simulink model "azmayeshe_AC_source"  (R2015a)
settings: Solver=ode45  StartTime=0.02  StopTime=0.04  RelTol=1e-3
libraries: powerlib x44, simulink x14, powerlib_meascontrol x14
settings Model: Creator=Yahya  LastModifiedBy=Yahya

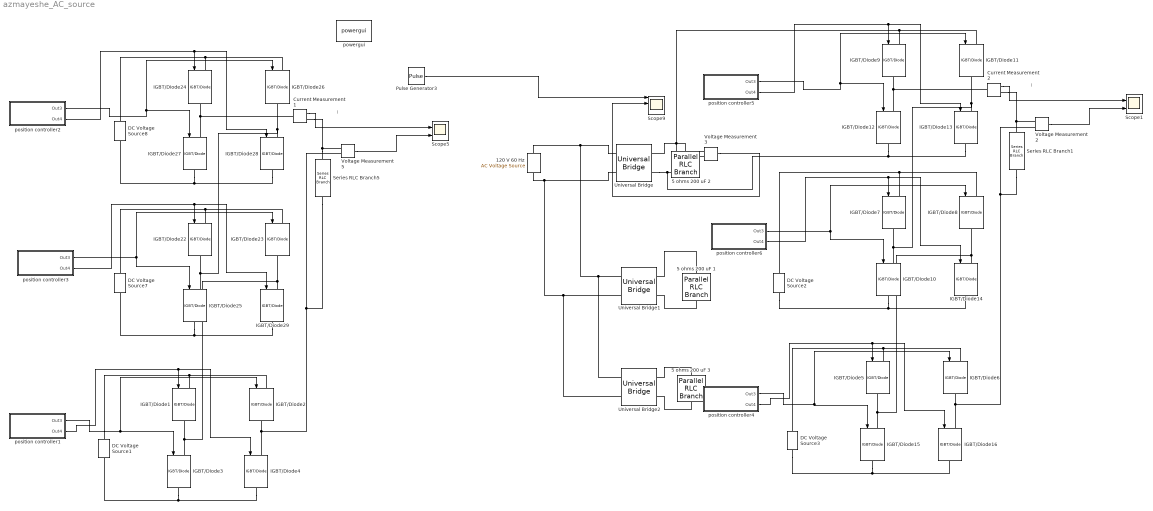
== system azmayeshe_AC_source ==
  note: i
  note: i
  120 V 60 Hz : powerlib/Electrical Sources/AC Voltage Source  Description=source block  Amplitude=100  Phase=0  Frequency=60  SampleTime=0  Measurements=None
      settings: AttributesFormatString=\n
  5 ohms 200 uF 1 : powerlib/Elements/Parallel RLC Branch  LConnTagsString=a  RConnTagsString=__new0  BranchType=C  Resistance=5  Inductance=1.0  SetiL0=off  InitialCurrent=0  Capacitance=470e-06  Setx0=off  InitialVoltage=0  Measurements=None
  5 ohms 200 uF 2 : powerlib/Elements/Parallel RLC Branch  LConnTagsString=a  RConnTagsString=__new0  BranchType=C  Resistance=5  Inductance=1.0  SetiL0=off  InitialCurrent=0  Capacitance=470e-06  Setx0=off  InitialVoltage=0  Measurements=None
  5 ohms 200 uF 3 : powerlib/Elements/Parallel RLC Branch  LConnTagsString=a  RConnTagsString=__new0  BranchType=C  Resistance=5  Inductance=1.0  SetiL0=off  InitialCurrent=0  Capacitance=470e-06  Setx0=off  InitialVoltage=0  Measurements=None
  Current Measurement1 : powerlib/Measurements/Current Measurement  PhasorSimulation=off  OutputType=Complex  PSBequivalent=0
  Current Measurement2 : powerlib/Measurements/Current Measurement  PhasorSimulation=off  OutputType=Complex  PSBequivalent=0
  DC Voltage Source{1..3,7..8} (5 alike) : powerlib/Electrical Sources/DC Voltage Source  Amplitude=100  Measurements=None
  IGBT/Diode{1..16,22..29} (24 alike) : powerlib/Power Electronics/IGBT//Diode  Ron=1e-3  Rs=1e5  Cs=inf  Measurements=off
  Pulse Generator3 : DiscretePulseGenerator  PulseType=Time based  Amplitude=0.8  Period=0.00001  PulseWidth=50
  Scope1 : Scope  NumInputPorts=2
      settings: TimeRange=1  YMin=-400~-400  YMax=400~400  SaveName=ScopeData2
  Scope5 : Scope  NumInputPorts=2
      settings: TimeRange=1  YMin=-400~-400  YMax=400~400  SaveName=ScopeData3
  Scope9 : Scope  NumInputPorts=4
      settings: YMin=-5~-5~-5~-5  YMax=5~5~5~5  SaveName=ScopeData18
  Series RLC Branch1 : powerlib/Elements/Series RLC Branch  LConnTagsString=__new0  RConnTagsString=__new0  BranchType=R  Resistance=1  Inductance=1e-5  SetiL0=off  InitialCurrent=0  Capacitance=1e-6  Setx0=off  InitialVoltage=0  Measurements=None
  Series RLC Branch5 : powerlib/Elements/Series RLC Branch  LConnTagsString=__new0  RConnTagsString=__new0  BranchType=R  Resistance=1  Inductance=1e-5  SetiL0=off  InitialCurrent=0  Capacitance=1e-6  Setx0=off  InitialVoltage=0  Measurements=None
  Universal Bridge : powerlib/Power Electronics/Universal Bridge  Arms=2  SnubberResistance=250  SnubberCapacitance=0.1e-6  Device=Diodes  Ron=0.01  Lon=0  ForwardVoltages="[  0.8  0.8  ]"  ForwardVoltage=0.8  GTOparameters=[ 10e-6 , 20e-6 ]  IGBTparameters=[ 1e-6 , 2e-6 ]  Measurements=Device currents  Measurements_2=None  converterType=Rectifier
  Universal Bridge1 : powerlib/Power Electronics/Universal Bridge  Arms=2  SnubberResistance=250  SnubberCapacitance=0.1e-6  Device=Diodes  Ron=0.01  Lon=0  ForwardVoltages="[  0.8  0.8  ]"  ForwardVoltage=0.8  GTOparameters=[ 10e-6 , 20e-6 ]  IGBTparameters=[ 1e-6 , 2e-6 ]  Measurements=Device currents  Measurements_2=None  converterType=Rectifier
  Universal Bridge2 : powerlib/Power Electronics/Universal Bridge  Arms=2  SnubberResistance=250  SnubberCapacitance=0.1e-6  Device=Diodes  Ron=0.01  Lon=0  ForwardVoltages="[  0.8  0.8  ]"  ForwardVoltage=0.8  GTOparameters=[ 10e-6 , 20e-6 ]  IGBTparameters=[ 1e-6 , 2e-6 ]  Measurements=Device currents  Measurements_2=None  converterType=Rectifier
  Voltage Measurement2 : powerlib/Measurements/Voltage Measurement  PhasorSimulation=off  OutputType=Complex  PSBequivalent=0
  Voltage Measurement3 : powerlib/Measurements/Voltage Measurement  PhasorSimulation=off  OutputType=Complex  PSBequivalent=0
  Voltage Measurement5 : powerlib/Measurements/Voltage Measurement  PhasorSimulation=off  OutputType=Complex  PSBequivalent=0
  position controller1 : Subsystem
  position controller2 : Subsystem
  position controller3 : Subsystem
  position controller4 : Subsystem
  position controller5 : Subsystem
  position controller6 : Subsystem
  powergui : powerlib/powergui  Priority=1  SimulationMode=Continuous  SolverType=Tustin/Backward Euler (TBE)  SampleTime=50e-6  frequency=60  SPID=off  DisableSnubberDevices=off  DisableRonSwitches=off  DisableVfSwitches=off  SwTol=0  DisplayEquations=off  Interpol=off  methode=off  Ts=100  FunctionMessages=off  echomessages=off  HookPort=off  EnableUseOfTLC=off  x0status=blocks  frequencyindice=0  Pbase=100e6  ErrMax=1e-4  Iterations=50  UnitsV=kV  UnitsW=MW  buscounter=0  RestoreLinks=warning  ResistiveCurrentMeasurement=off  Frange=[0:2:500]  Ylog=off  Xlog=on  ShowGrid=off  save=off  variable=ZData  structure=0  ZoomFFT=off  StartTime=0.0  cycles=1  DisplayStyle=1  fundamental=60  FreqAxis=off  MaxFrequency=1000  frequencyindicesteady=1  RmsSteady=1  display=off
  wires:
  position controller2/2(Out4) -> IGBT/Diode28/1, IGBT/Diode24/1
  position controller2/1(Out3) -> IGBT/Diode26/1, IGBT/Diode27/1
  position controller3/2(Out4) -> IGBT/Diode29/1, IGBT/Diode22/1
  position controller3/1(Out3) -> IGBT/Diode23/1, IGBT/Diode25/1
  Current Measurement1/1 -> Scope5/1
  position controller1/2(Out4) -> IGBT/Diode4/1, IGBT/Diode1/1
  position controller1/1(Out3) -> IGBT/Diode3/1, IGBT/Diode2/1
  Voltage Measurement5/1 -> Scope5/2
  Pulse Generator3/1 -> Scope9/1
  position controller5/2(Out4) -> IGBT/Diode13/1, IGBT/Diode9/1
  position controller5/1(Out3) -> IGBT/Diode11/1, IGBT/Diode12/1
  position controller6/2(Out4) -> IGBT/Diode14/1, IGBT/Diode7/1
  position controller6/1(Out3) -> IGBT/Diode8/1, IGBT/Diode10/1
  Current Measurement2/1 -> Scope1/1
  position controller4/2(Out4) -> IGBT/Diode16/1, IGBT/Diode5/1
  position controller4/1(Out3) -> IGBT/Diode15/1, IGBT/Diode6/1
  Voltage Measurement2/1 -> Scope1/2
  Voltage Measurement3/1 -> Scope9/2
  connections:
  IGBT/Diode26/LConn1 -- IGBT/Diode24/LConn1 -- DC Voltage Source8/RConn1
  IGBT/Diode27/RConn1 -- IGBT/Diode28/RConn1 -- DC Voltage Source8/LConn1
  IGBT/Diode27/LConn1 -- Current Measurement1/LConn1 -- IGBT/Diode24/RConn1
  IGBT/Diode23/LConn1 -- IGBT/Diode22/LConn1 -- DC Voltage Source7/RConn1
  IGBT/Diode29/RConn1 -- IGBT/Diode25/RConn1 -- DC Voltage Source7/LConn1
  IGBT/Diode25/LConn1 -- IGBT/Diode22/RConn1 -- IGBT/Diode26/RConn1 -- IGBT/Diode28/LConn1
  IGBT/Diode23/RConn1 -- IGBT/Diode29/LConn1 -- IGBT/Diode1/RConn1 -- IGBT/Diode3/LConn1
  Series RLC Branch5/LConn1 -- Current Measurement1/RConn1 -- Voltage Measurement5/LConn1
  DC Voltage Source1/RConn1 -- IGBT/Diode2/LConn1 -- IGBT/Diode1/LConn1
  DC Voltage Source1/LConn1 -- IGBT/Diode4/RConn1 -- IGBT/Diode3/RConn1
  Voltage Measurement5/LConn2 -- Series RLC Branch5/RConn1 -- IGBT/Diode2/RConn1 -- IGBT/Diode4/LConn1
  IGBT/Diode9/LConn1 -- Voltage Measurement3/LConn1 -- Universal Bridge/RConn1 -- 5 ohms 200 uF 2/LConn1 -- IGBT/Diode11/LConn1
  120 V 60 Hz/LConn1 -- Universal Bridge2/LConn2 -- Universal Bridge1/LConn2 -- Universal Bridge/LConn2
  120 V 60 Hz/RConn1 -- Universal Bridge2/LConn1 -- Universal Bridge1/LConn1 -- Universal Bridge/LConn1
  IGBT/Diode13/RConn1 -- Voltage Measurement3/LConn2 -- 5 ohms 200 uF 2/RConn1 -- Universal Bridge/RConn2 -- IGBT/Diode12/RConn1
  IGBT/Diode9/RConn1 -- IGBT/Diode12/LConn1 -- Current Measurement2/LConn1
  IGBT/Diode7/RConn1 -- IGBT/Diode10/LConn1 -- IGBT/Diode11/RConn1 -- IGBT/Diode13/LConn1
  IGBT/Diode14/LConn1 -- IGBT/Diode8/RConn1 -- IGBT/Diode5/RConn1 -- IGBT/Diode15/LConn1
  Voltage Measurement2/LConn1 -- Current Measurement2/RConn1 -- Series RLC Branch1/LConn1
  IGBT/Diode16/LConn1 -- Series RLC Branch1/RConn1 -- Voltage Measurement2/LConn2 -- IGBT/Diode6/RConn1
  IGBT/Diode7/LConn1 -- IGBT/Diode8/LConn1 -- DC Voltage Source2/RConn1
  IGBT/Diode10/RConn1 -- IGBT/Diode14/RConn1 -- DC Voltage Source2/LConn1
  IGBT/Diode5/LConn1 -- IGBT/Diode6/LConn1 -- DC Voltage Source3/RConn1
  IGBT/Diode15/RConn1 -- DC Voltage Source3/LConn1 -- IGBT/Diode16/RConn1
  5 ohms 200 uF 1/RConn1 -- Universal Bridge1/RConn2
  5 ohms 200 uF 1/LConn1 -- Universal Bridge1/RConn1
  5 ohms 200 uF 3/RConn1 -- Universal Bridge2/RConn2
  5 ohms 200 uF 3/LConn1 -- Universal Bridge2/RConn1

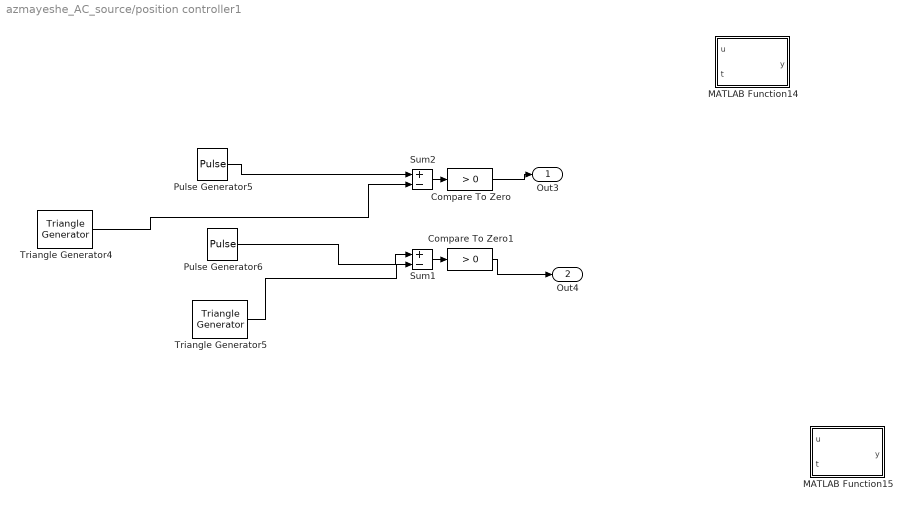
== system azmayeshe_AC_source/position controller1 ==
  Compare To Zero : simulink/Logic and Bit Operations/Compare To Zero  relop=>  OutDataTypeStr=boolean  ZeroCross=off
  Compare To Zero1 : simulink/Logic and Bit Operations/Compare To Zero  relop=>  OutDataTypeStr=boolean  ZeroCross=off
  MATLAB Function14 : MATLAB Function  TreatAsAtomicUnit=on
  MATLAB Function15 : MATLAB Function  TreatAsAtomicUnit=on
  Pulse Generator5 : DiscretePulseGenerator  PulseType=Time based  Amplitude=0.1254  Period=0.02  PulseWidth=50.001
  Pulse Generator6 : DiscretePulseGenerator  PulseType=Time based  Amplitude=0.1254  Period=0.02  PulseWidth=50.001  PhaseDelay=0.01
  Sum1 : Sum  Inputs=+-  OutDataTypeStr=double
  Sum2 : Sum  Inputs=+-  OutDataTypeStr=double
  Triangle Generator4 : powerlib_meascontrol/Pulse & Signal Generators/Triangle Generator  Freq=50  Phase=90  Ts=0
  Triangle Generator5 : powerlib_meascontrol/Pulse & Signal Generators/Triangle Generator  Freq=50  Phase=90+180  Ts=0
  Out3 : Outport
  Out4 : Outport  Port=2
  wires:
  Compare To Zero/1 -> Out3/1
  Compare To Zero1/1 -> Out4/1
  Triangle Generator4/1 -> Sum2/2
  Sum2/1 -> Compare To Zero/1
  Sum1/1 -> Compare To Zero1/1
  Pulse Generator5/1 -> Sum2/1
  Pulse Generator6/1 -> Sum1/1
  Triangle Generator5/1 -> Sum1/2

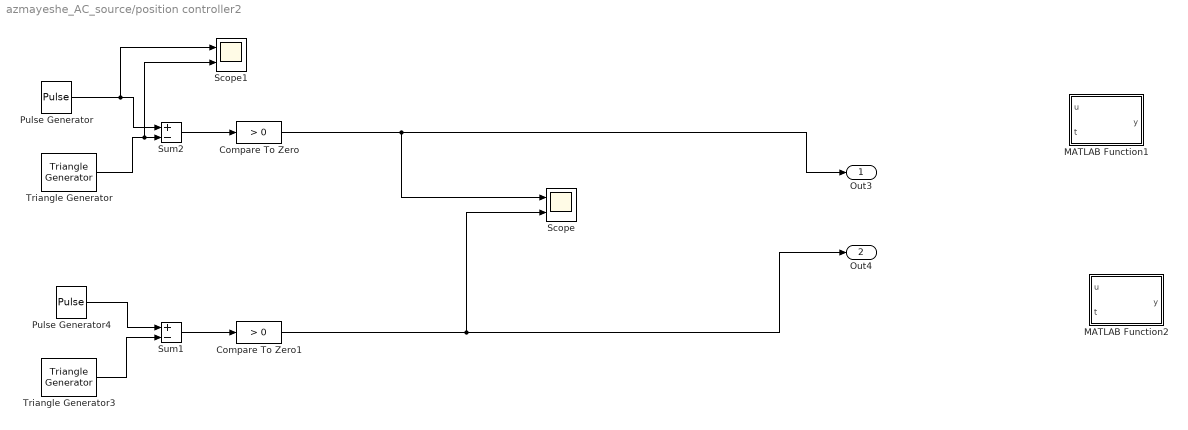
== system azmayeshe_AC_source/position controller2 ==
  Compare To Zero : simulink/Logic and Bit Operations/Compare To Zero  relop=>  OutDataTypeStr=boolean  ZeroCross=off
  Compare To Zero1 : simulink/Logic and Bit Operations/Compare To Zero  relop=>  OutDataTypeStr=boolean  ZeroCross=off
  MATLAB Function1 : MATLAB Function  TreatAsAtomicUnit=on
  MATLAB Function2 : MATLAB Function  TreatAsAtomicUnit=on
  Pulse Generator : DiscretePulseGenerator  PulseType=Time based  Amplitude=0.6526  Period=0.02  PulseWidth=50.001
  Pulse Generator4 : DiscretePulseGenerator  PulseType=Time based  Amplitude=0.6526  Period=0.02  PulseWidth=50.001  PhaseDelay=0.01
  Scope : Scope  NumInputPorts=2
      settings: YMin=-5~-5  YMax=5~5
  Scope1 : Scope  NumInputPorts=2
      settings: YMin=-5~-5  YMax=5~5
  Sum1 : Sum  Inputs=+-  OutDataTypeStr=double
  Sum2 : Sum  Inputs=+-  OutDataTypeStr=double
  Triangle Generator : powerlib_meascontrol/Pulse & Signal Generators/Triangle Generator  Freq=50  Phase=90  Ts=0
  Triangle Generator3 : powerlib_meascontrol/Pulse & Signal Generators/Triangle Generator  Freq=50  Phase=90+180  Ts=0
  Out3 : Outport
  Out4 : Outport  Port=2
  wires:
  Pulse Generator/1 -> Scope1/1, Sum2/1
  Triangle Generator/1 -> Scope1/2, Sum2/2
  Pulse Generator4/1 -> Sum1/1
  Triangle Generator3/1 -> Sum1/2
  Compare To Zero1/1 -> Scope/2, Out4/1
  Sum2/1 -> Compare To Zero/1
  Sum1/1 -> Compare To Zero1/1
  Compare To Zero/1 -> Scope/1, Out3/1

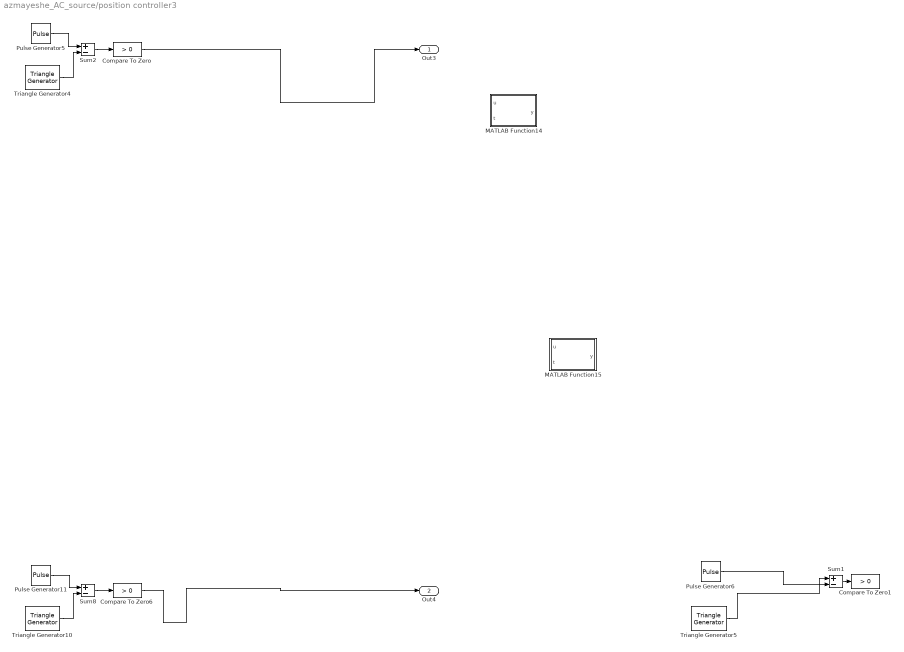
== system azmayeshe_AC_source/position controller3 ==
  Compare To Zero : simulink/Logic and Bit Operations/Compare To Zero  relop=>  OutDataTypeStr=boolean  ZeroCross=off
  Compare To Zero1 : simulink/Logic and Bit Operations/Compare To Zero  relop=>  OutDataTypeStr=boolean  ZeroCross=off
  Compare To Zero6 : simulink/Logic and Bit Operations/Compare To Zero  relop=>  OutDataTypeStr=boolean  ZeroCross=off
  MATLAB Function14 : MATLAB Function  TreatAsAtomicUnit=on
  MATLAB Function15 : MATLAB Function  TreatAsAtomicUnit=on
  Pulse Generator11 : DiscretePulseGenerator  PulseType=Time based  Amplitude=0.3487  Period=0.02  PulseWidth=50.001  PhaseDelay=0.01
  Pulse Generator5 : DiscretePulseGenerator  PulseType=Time based  Amplitude=0.3487  Period=0.02  PulseWidth=50.001
  Pulse Generator6 : DiscretePulseGenerator  PulseType=Time based  Amplitude=0.332  Period=0.02  PulseWidth=50  PhaseDelay=0.01
  Sum1 : Sum  Inputs=+-  OutDataTypeStr=double
  Sum2 : Sum  Inputs=+-  OutDataTypeStr=double
  Sum8 : Sum  Inputs=+-  OutDataTypeStr=double
  Triangle Generator10 : powerlib_meascontrol/Pulse & Signal Generators/Triangle Generator  Freq=50  Phase=90+180  Ts=0
  Triangle Generator4 : powerlib_meascontrol/Pulse & Signal Generators/Triangle Generator  Freq=50  Phase=90  Ts=0
  Triangle Generator5 : powerlib_meascontrol/Pulse & Signal Generators/Triangle Generator  Freq=50  Phase=90+180  Ts=0
  Out3 : Outport
  Out4 : Outport  Port=2
  wires:
  Triangle Generator4/1 -> Sum2/2
  Sum2/1 -> Compare To Zero/1
  Sum1/1 -> Compare To Zero1/1
  Pulse Generator5/1 -> Sum2/1
  Pulse Generator6/1 -> Sum1/1
  Triangle Generator5/1 -> Sum1/2
  Compare To Zero/1 -> Out3/1
  Triangle Generator10/1 -> Sum8/2
  Sum8/1 -> Compare To Zero6/1
  Pulse Generator11/1 -> Sum8/1
  Compare To Zero6/1 -> Out4/1

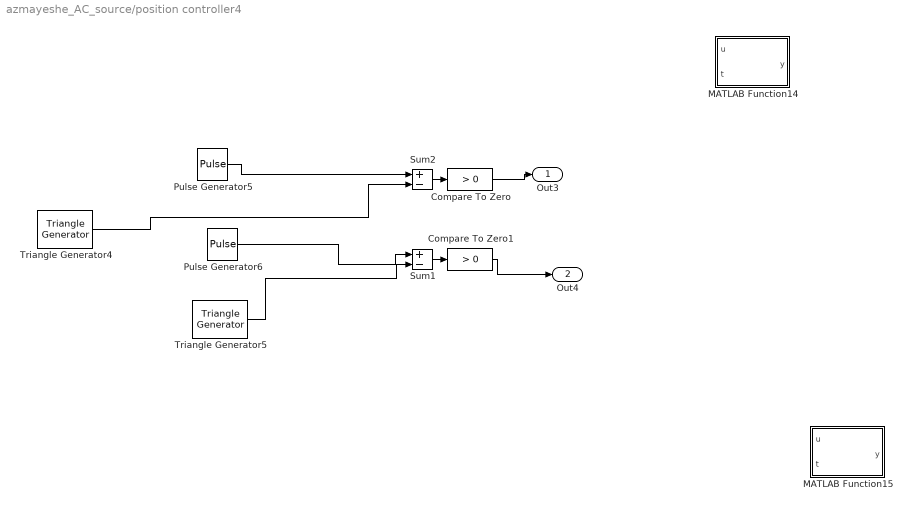
== system azmayeshe_AC_source/position controller4 ==
  Compare To Zero : simulink/Logic and Bit Operations/Compare To Zero  relop=>  OutDataTypeStr=boolean  ZeroCross=off
  Compare To Zero1 : simulink/Logic and Bit Operations/Compare To Zero  relop=>  OutDataTypeStr=boolean  ZeroCross=off
  MATLAB Function14 : MATLAB Function  TreatAsAtomicUnit=on
  MATLAB Function15 : MATLAB Function  TreatAsAtomicUnit=on
  Pulse Generator5 : DiscretePulseGenerator  PulseType=Time based  Amplitude=0.1254  Period=0.02  PulseWidth=50.001
  Pulse Generator6 : DiscretePulseGenerator  PulseType=Time based  Amplitude=0.1254  Period=0.02  PulseWidth=50.001  PhaseDelay=0.01
  Sum1 : Sum  Inputs=+-  OutDataTypeStr=double
  Sum2 : Sum  Inputs=+-  OutDataTypeStr=double
  Triangle Generator4 : powerlib_meascontrol/Pulse & Signal Generators/Triangle Generator  Freq=50  Phase=90  Ts=0
  Triangle Generator5 : powerlib_meascontrol/Pulse & Signal Generators/Triangle Generator  Freq=50  Phase=90+180  Ts=0
  Out3 : Outport
  Out4 : Outport  Port=2
  wires:
  Compare To Zero/1 -> Out3/1
  Compare To Zero1/1 -> Out4/1
  Triangle Generator4/1 -> Sum2/2
  Sum2/1 -> Compare To Zero/1
  Sum1/1 -> Compare To Zero1/1
  Pulse Generator5/1 -> Sum2/1
  Pulse Generator6/1 -> Sum1/1
  Triangle Generator5/1 -> Sum1/2

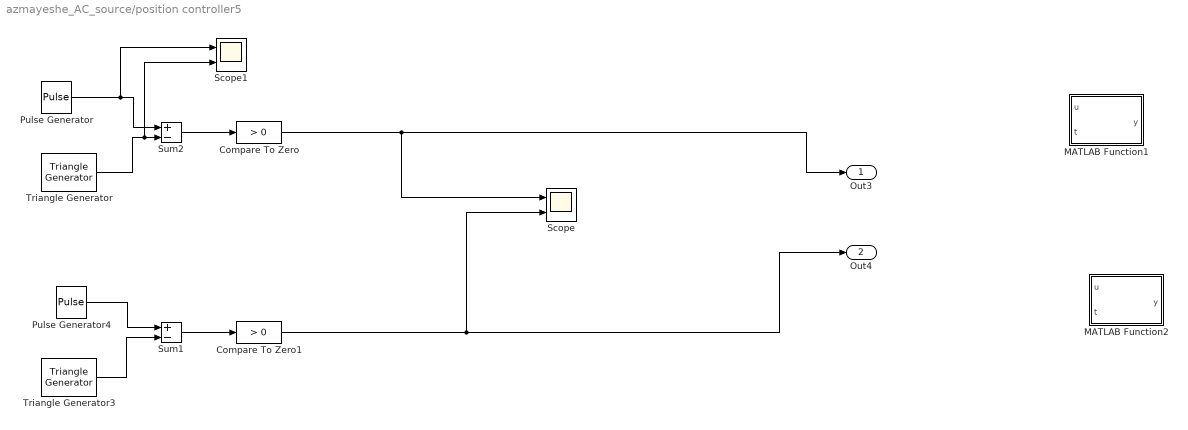
== system azmayeshe_AC_source/position controller5 ==
  Compare To Zero : simulink/Logic and Bit Operations/Compare To Zero  relop=>  OutDataTypeStr=boolean  ZeroCross=off
  Compare To Zero1 : simulink/Logic and Bit Operations/Compare To Zero  relop=>  OutDataTypeStr=boolean  ZeroCross=off
  MATLAB Function1 : MATLAB Function  TreatAsAtomicUnit=on
  MATLAB Function2 : MATLAB Function  TreatAsAtomicUnit=on
  Pulse Generator : DiscretePulseGenerator  PulseType=Time based  Amplitude=0.6526  Period=0.02  PulseWidth=50.001
  Pulse Generator4 : DiscretePulseGenerator  PulseType=Time based  Amplitude=0.6526  Period=0.02  PulseWidth=50.001  PhaseDelay=0.01
  Scope : Scope  NumInputPorts=2
      settings: YMin=-5~-5  YMax=5~5
  Scope1 : Scope  NumInputPorts=2
      settings: YMin=-5~-5  YMax=5~5
  Sum1 : Sum  Inputs=+-  OutDataTypeStr=double
  Sum2 : Sum  Inputs=+-  OutDataTypeStr=double
  Triangle Generator : powerlib_meascontrol/Pulse & Signal Generators/Triangle Generator  Freq=50  Phase=90  Ts=0
  Triangle Generator3 : powerlib_meascontrol/Pulse & Signal Generators/Triangle Generator  Freq=50  Phase=90+180  Ts=0
  Out3 : Outport
  Out4 : Outport  Port=2
  wires:
  Pulse Generator/1 -> Scope1/1, Sum2/1
  Triangle Generator/1 -> Scope1/2, Sum2/2
  Pulse Generator4/1 -> Sum1/1
  Triangle Generator3/1 -> Sum1/2
  Compare To Zero1/1 -> Scope/2, Out4/1
  Sum2/1 -> Compare To Zero/1
  Sum1/1 -> Compare To Zero1/1
  Compare To Zero/1 -> Scope/1, Out3/1

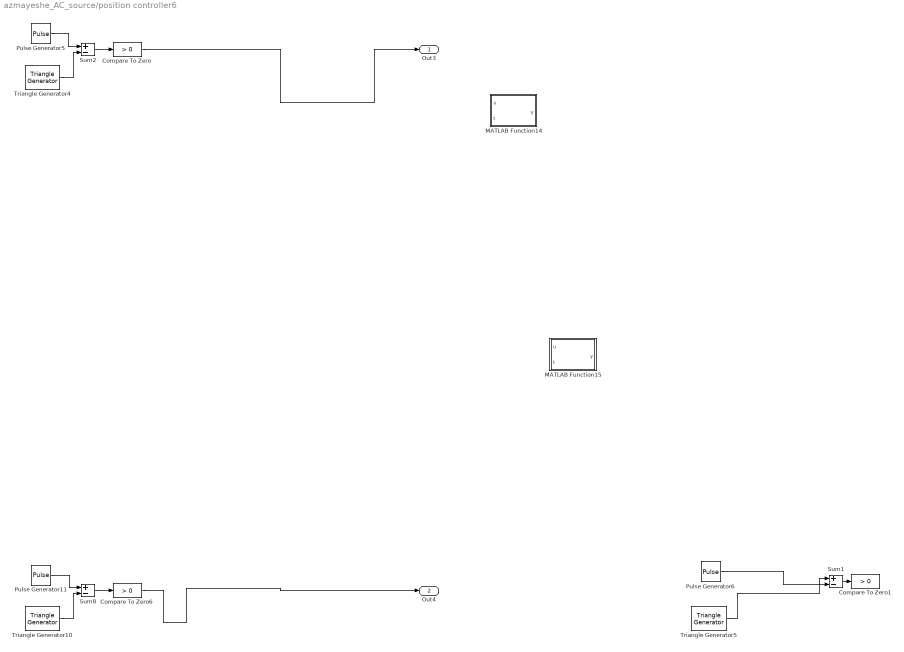
== system azmayeshe_AC_source/position controller6 ==
  Compare To Zero : simulink/Logic and Bit Operations/Compare To Zero  relop=>  OutDataTypeStr=boolean  ZeroCross=off
  Compare To Zero1 : simulink/Logic and Bit Operations/Compare To Zero  relop=>  OutDataTypeStr=boolean  ZeroCross=off
  Compare To Zero6 : simulink/Logic and Bit Operations/Compare To Zero  relop=>  OutDataTypeStr=boolean  ZeroCross=off
  MATLAB Function14 : MATLAB Function  TreatAsAtomicUnit=on
  MATLAB Function15 : MATLAB Function  TreatAsAtomicUnit=on
  Pulse Generator11 : DiscretePulseGenerator  PulseType=Time based  Amplitude=0.3487  Period=0.02  PulseWidth=50.001  PhaseDelay=0.01
  Pulse Generator5 : DiscretePulseGenerator  PulseType=Time based  Amplitude=0.3487  Period=0.02  PulseWidth=50.001
  Pulse Generator6 : DiscretePulseGenerator  PulseType=Time based  Amplitude=0.332  Period=0.02  PulseWidth=50  PhaseDelay=0.01
  Sum1 : Sum  Inputs=+-  OutDataTypeStr=double
  Sum2 : Sum  Inputs=+-  OutDataTypeStr=double
  Sum8 : Sum  Inputs=+-  OutDataTypeStr=double
  Triangle Generator10 : powerlib_meascontrol/Pulse & Signal Generators/Triangle Generator  Freq=50  Phase=90+180  Ts=0
  Triangle Generator4 : powerlib_meascontrol/Pulse & Signal Generators/Triangle Generator  Freq=50  Phase=90  Ts=0
  Triangle Generator5 : powerlib_meascontrol/Pulse & Signal Generators/Triangle Generator  Freq=50  Phase=90+180  Ts=0
  Out3 : Outport
  Out4 : Outport  Port=2
  wires:
  Triangle Generator4/1 -> Sum2/2
  Sum2/1 -> Compare To Zero/1
  Sum1/1 -> Compare To Zero1/1
  Pulse Generator5/1 -> Sum2/1
  Pulse Generator6/1 -> Sum1/1
  Triangle Generator5/1 -> Sum1/2
  Compare To Zero/1 -> Out3/1
  Triangle Generator10/1 -> Sum8/2
  Sum8/1 -> Compare To Zero6/1
  Pulse Generator11/1 -> Sum8/1
  Compare To Zero6/1 -> Out4/1

== matlab function azmayeshe_AC_source/position controller3/MATLAB Function14 ==
  data: u input; y output; t input
function y = fcn(u,t)
%#codegen
if t>u
    y = 1;
else
    y = 0;
end
end

== matlab function azmayeshe_AC_source/position controller4/MATLAB Function14 ==
  data: u input; y output; t input
function y = fcn(u,t)
%#codegen
if t>u
    y = 1;
else
    y = 0;
end
end

== matlab function azmayeshe_AC_source/position controller1/MATLAB Function14 ==
  data: u input; y output; t input
function y = fcn(u,t)
%#codegen
if t>u
    y = 1;
else
    y = 0;
end
end

== matlab function azmayeshe_AC_source/position controller4/MATLAB Function15 ==
  data: u input; y output; t input
function y = fcn(u,t)
%#codegen
if t>u
    y = 1;
else
    y = 0;
end
end

== matlab function azmayeshe_AC_source/position controller2/MATLAB Function1 ==
  data: u input; y output; t input
function y = fcn(u,t)
%#codegen
if t>u
    y = 1;
else
    y = 0;
end
end

== matlab function azmayeshe_AC_source/position controller2/MATLAB Function2 ==
  data: u input; y output; t input
function y = fcn(u,t)
%#codegen
if t>u
    y = 1;
else
    y = 0;
end
end

== matlab function azmayeshe_AC_source/position controller1/MATLAB Function15 ==
  data: u input; y output; t input
function y = fcn(u,t)
%#codegen
if t>u
    y = 1;
else
    y = 0;
end
end

== matlab function azmayeshe_AC_source/position controller5/MATLAB Function1 ==
  data: u input; y output; t input
function y = fcn(u,t)
%#codegen
if t>u
    y = 1;
else
    y = 0;
end
end

== matlab function azmayeshe_AC_source/position controller5/MATLAB Function2 ==
  data: u input; y output; t input
function y = fcn(u,t)
%#codegen
if t>u
    y = 1;
else
    y = 0;
end
end

== matlab function azmayeshe_AC_source/position controller6/MATLAB Function14 ==
  data: u input; y output; t input
function y = fcn(u,t)
%#codegen
if t>u
    y = 1;
else
    y = 0;
end
end

== matlab function azmayeshe_AC_source/position controller6/MATLAB Function15 ==
  data: u input; y output; t input
function y = fcn(u,t)
%#codegen
if t>u
    y = 1;
else
    y = 0;
end
end

== matlab function azmayeshe_AC_source/position controller3/MATLAB Function15 ==
  data: u input; y output; t input
function y = fcn(u,t)
%#codegen
if t>u
    y = 1;
else
    y = 0;
end
end
